simulink model "atrias_system_4khz"  (R2016b)
settings: Solver=FixedStepDiscrete  StartTime=0.0  StopTime=inf  FixedStep=elmo_sample_time  RelTol=1e-3
undefined symbols (not defined in the file or in its folder): gui_disable_cmd, gui_enable_cmd, gui_exit_cmd, gui_reset_cmd, HARD_MOTOR_POSITION_LIMITS_LOWER, HARD_MOTOR_POSITION_LIMITS_UPPER, HIP_ABS_MAX_ENCODER_TICKS, HIP_CURRENT_LIMIT, HIP_INC_MAX_ENCODER_TICKS, HIP_MOTOR_CONSTANT, HIP_MTR_GEAR_RATIO, HIP_MTR_MAX_TORQUE, LEFT_MOTOR_HIP_DIRECTION, LEG1_MOTOR_A_DIRECTION, LEG1_MOTOR_B_DIRECTION, LEG2_MOTOR_A_DIRECTION, LEG2_MOTOR_B_DIRECTION, LEG_CURRENT_LIMIT, LEG_INC_ENCODER_DIRECTION_LEFT_BACK, LEG_INC_ENCODER_DIRECTION_LEFT_FRONT, LEG_INC_ENCODER_DIRECTION_RIGHT_BACK, LEG_INC_ENCODER_DIRECTION_RIGHT_FRONT, LEG_INC_ENCODER_RAD_PER_TICK, LEG_MOTOR_CONSTANT, LEG_MTR_GEAR_RATIO, LEG_MTR_MAX_TORQUE, max_hip_velocity, max_motor_velocity, MEDULLA_ADC_MAX_VOLTS, MEDULLA_ADC_OFFSET_COUNTS, MEDULLA_STATE_ERROR, MEDULLA_STATE_HALT, MEDULLA_STATE_IDLE, MEDULLA_STATE_RESET, MEDULLA_STATE_RUN, MOTOR_POSITION_LIMITS_LOWER, MOTOR_POSITION_LIMITS_UPPER, MTR_HIP_MAX_CURRENT, MTR_MAX_CONT_CURRENT, MTR_MAX_COUNT, MTR_MAX_CURRENT, MTR_MAX_TEMP, RIGHT_MOTOR_HIP_DIRECTION
libraries: xpcethercatlib x190, simulink x37
(part 1 of 4)
settings Model: xpc_rtwmakecfg_data=_xpcethercatlib_  SimulationMode=external  ParamWorkspaceSource=ReferencedWorkspace  Creator=wmartin  LastModifiedBy=Will
settings SolverCC: EnableConcurrentExecution=on
settings DataIOCC: LimitDataPoints=on  MaxDataPoints=1000000000  SaveFormat=StructureWithTime  SaveOutput=off  SaveTime=off
settings OptimizationCC: BlockReduction=off  DefaultParameterBehavior=Inlined  OptimizeBlockIOStorage=off  BufferReuse=off  GlobalBufferReuse=off  ExpressionFolding=off  ExpressionDepthLimit=2147483647  LocalBlockOutputs=off  LifeSpan=inf  SimCompilerOptimization=on
settings DebuggingCC: UnderspecifiedInitializationDetection=Classic  MergeDetectMultiDrivingBlocksExec=none  SolverPrmCheckMsg=warning  StateNameClashWarn=warning  SFUnexpectedBacktrackingDiag=warning  SFNoUnconditionalDefaultTransitionDiag=warning  SFExecutionAtInitializationDiag=none
settings HardwareCC: ProdBitPerPointer=32  ProdBitPerSizeT=32  ProdBitPerPtrDiffT=32  ProdLargestAtomicFloat=None  ProdWordSize=32  ProdLongLongMode=on  ProdHWDeviceType=Generic->32-bit x86 compatible
settings ModelReferenceCC: EnableParallelModelReferenceBuilds=on  ModelReferenceNumInstancesAllowed=Single  ModelReferenceMinAlgLoopOccurrences=on  PropagateSignalLabelsOutOfModel=off
settings RTWCC: SystemTargetFile=slrt.tlc  TemplateMakefile=slrt_default_tmf  Description=Simulink Real-Time  RTWVerbose=off  RTWCompilerOptimization=on
settings CodeAppCC: MaxIdLength=256
settings SimulinkRealTimeCC: GeneratePreprocessorConditionals=Disable all  RL32LogBufSizeModifier=100000000
settings ConfigComp: CovMetricSettings=dw  CovHtmlReporting=on  CovSaveCumulativeToWorkspaceVar=on  CovSaveSingleToWorkspaceVar=on  CovExternalEMLEnable=off  CovSFcnEnable=off

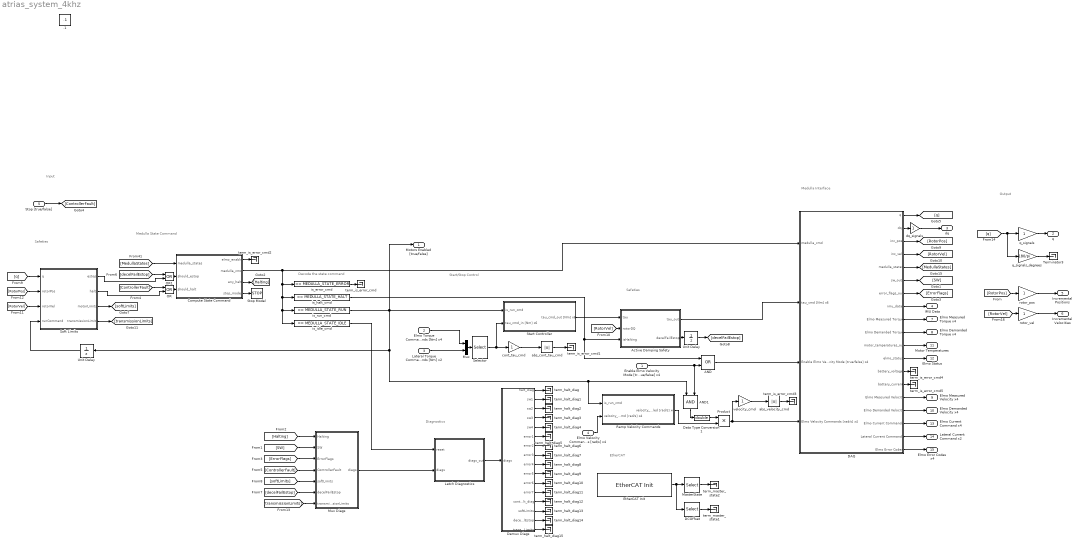
== system atrias_system_4khz ==
  note: Decode the state command
  note: Medulla Interface
  note: Medulla State Command
  note: Diagnostics
  note: EtherCAT
  note: Start/Stop Control
  note: Input
  note: Safeties
  note: Safeties
  note: Output
  Enable Elmo Velocity Mode [true/false] x4 : Inport  OutDataTypeStr=boolean  PortDimensions=4
  Elmo Torque Commands [Nm] x4 : Inport  Port=2  PortDimensions=4
  Lateral Torque Commands [Nm] x2 : Inport  Port=3  PortDimensions=2
  Elmo Velocity Commands [rad/s] x4 : Inport  Port=4  OutDataTypeStr=double  PortDimensions=4
  Stop [true/false] : Inport  Port=5  OutDataTypeStr=boolean
  AND : Logic  Operator=OR  AllPortsSameDT=off  OutDataTypeStr=boolean
  AND1 : Logic  AllPortsSameDT=off  OutDataTypeStr=boolean
  Active Damping Safety : MATLAB Function  TreatAsAtomicUnit=on
  Compute State Command : MATLAB Function  TreatAsAtomicUnit=on
  DAQ : Subsystem
  DCOffset : Selector  InputPortWidth=6  IndexOptions=Index vector (dialog)  Indices=[4]  OutputSizes=1
  Data Type Conversion1 : DataTypeConversion  OutDataTypeStr=double
  Demux Diags : MATLAB Function  TreatAsAtomicUnit=on
  EtherCAT Init : xpcethercatlib/EtherCAT Init   Priority=0  config_file=7medullas4emlos_09_19_2016_4khz.xml  device_id=0  pci_bus=2  pci_slot=0  dctuning=0  enaDebug=off  enaDC=on  errLink=off  masterDbg=off  stateChgDbg=off  baseClock=off  masterCfg=off  logFile='E:\dbglog.txt'  sample_time=0.000250  DCMode=2
  Latch Diagnostics : MATLAB Function  TreatAsAtomicUnit=on
  MasterState : Selector  InputPortWidth=6  IndexOptions=Index vector (dialog)  Indices=[2]  OutputSizes=1
  Mux : Mux  Inputs=2
  Mux Diags : MATLAB Function  TreatAsAtomicUnit=on
  OR : Logic  Operator=OR  AllPortsSameDT=off  OutDataTypeStr=boolean
  OR1 : Logic  Operator=OR  AllPortsSameDT=off  OutDataTypeStr=boolean
  Product : Product
  Ramp Velocity Commands : Subsystem
  Selector : Selector  InputPortWidth=6  IndexOptions=Index vector (dialog)  Indices=[1 2 5 3 4 6]  OutputSizes=1
  Soft Limits : MATLAB Function  TreatAsAtomicUnit=on
  Start Controller : Subsystem
  Stop Model : Stop
  Terminator3 : Terminator
  Unit Delay : UnitDelay  SampleTime=-1
  "Unit Delay " : UnitDelay  SampleTime=-1
  abs_cont_tau_cmd : Abs
  abs_velocity_cmd : Abs
  cont_tau_cmd : Gain
  dq_signals : Gain
  is_error_cmd : simulink/Logic and Bit Operations/Compare To Constant  relop===  const=MEDULLA_STATE_ERROR  OutDataTypeStr=boolean
  is_halt_cmd : simulink/Logic and Bit Operations/Compare To Constant  relop===  const=MEDULLA_STATE_HALT  OutDataTypeStr=boolean
  is_idle_cmd : simulink/Logic and Bit Operations/Compare To Constant  relop===  const=MEDULLA_STATE_IDLE  OutDataTypeStr=boolean
  is_run_cmd : simulink/Logic and Bit Operations/Compare To Constant  relop===  const=MEDULLA_STATE_RUN  OutDataTypeStr=boolean
  q_signals : Gain
  q_signals_degrees : Gain  Gain=180/pi
  rotor_pos : Gain
  rotor_vel : Gain
  term_halt_diag{,1..15} (16 alike) : Terminator
  term_is_error_cmd{,1..5} (6 alike) : Terminator
  term_master_state1 : Terminator
  term_master_state2 : Terminator
  velocity_cmd : Gain
  Motors Enabled [true/false] : Outport
  q : Outport  Port=2
  dq : Outport  Port=3
  IMU Data : Outport  Port=4
  Incremental Positions : Outport  Port=5
  Incremental Velocities : Outport  Port=6
  Elmo Measured Torque x4 : Outport  Port=7
  Elmo Demanded Torque x4 : Outport  Port=8
  Elmo Measured Velocity x4 : Outport  Port=9
  Elmo Demanded Velocity x4 : Outport  Port=10
  Motor Temperatures : Outport  Port=11
  Elmo Status : Outport  Port=12
  Elmo Current Command x4 : Outport  Port=13
  Lateral Current Command x2 : Outport  Port=14
  Elmo Error Codes x4 : Outport  Port=15
  .1 : Constant  IOType=siggen  Value=.1
  wires:
  [MedullaStates] -> Compute State Command/1(medulla_states)
  Compute State Command/3(any_halt) -> [Halting]
  Latch Diagnostics/1(diags_out) -> Demux Diags/1(diags)
  is_error_cmd/1 -> term_is_error_cmd/1
  Selector/1 -> Start Controller/2(tau_cmd_in [Nm] x6), cont_tau_cmd/1
  Start Controller/1(tau_cmd_out [Nm] x6) -> Active Damping Safety/1(tau)
  is_idle_cmd/1 -> Latch Diagnostics/1(reset)
  DAQ/6(sw_out) -> [SW]
  Mux Diags/1(diags) -> Latch Diagnostics/2(diags)
  [Halting] -> Mux Diags/1(Halting)
  [SW] -> Mux Diags/2(SW)
  Demux Diags/2(sw1) -> term_halt_diag1/1
  Demux Diags/5(sw4) -> term_halt_diag4/1
  Demux Diags/4(sw3) -> term_halt_diag3/1
  Demux Diags/3(sw2) -> term_halt_diag2/1
  DAQ/7(error_flags_out) -> [ErrorFlags]
  [ErrorFlags] -> Mux Diags/3(ErrorFlags)
  Demux Diags/1(halt_diag) -> term_halt_diag/1
  Demux Diags/12(error7) -> term_halt_diag11/1
  Demux Diags/11(error6) -> term_halt_diag10/1
  Demux Diags/10(error5) -> term_halt_diag9/1
  Demux Diags/9(error4) -> term_halt_diag8/1
  Demux Diags/8(error3) -> term_halt_diag7/1
  Demux Diags/7(error2) -> term_halt_diag6/1
  Demux Diags/6(error1) -> term_halt_diag5/1
  abs_cont_tau_cmd/1 -> term_is_error_cmd1/1
  DAQ/8(imu_data) -> IMU Data/1
  [ControllerFault] -> Mux Diags/4(ControllerFault)
  Demux Diags/13(contrlr_fault_diag) -> term_halt_diag12/1
  [RotorPos] -> Soft Limits/2(rotorPos)
  [RotorVel] -> Soft Limits/3(rotorVel)
  EtherCAT Init/1 -> DCOffset/1, MasterState/1
  cont_tau_cmd/1 -> abs_cont_tau_cmd/1
  Stop [true/false]/1 -> [ControllerFault]
  [softLimits] -> Mux Diags/5(softLimits)
  Demux Diags/14(softLimits) -> term_halt_diag13/1
  Soft Limits/3(motorLimits) -> [softLimits]
  is_run_cmd/1 -> Start Controller/1(is_run_cmd), Motors Enabled [true/false]/1, Ramp Velocity Commands/1(is_run_cmd), AND1/1, Unit Delay/1
  Active Damping Safety/1(tau_out) -> DAQ/2(tau_cmd [Nm] x6)
  [RotorVel] -> Active Damping Safety/2(rotorDQ)
  DCOffset/1 -> term_master_state1/1
  [q] -> Soft Limits/1(q)
  [decelFailEstop] -> Mux Diags/6(decelFailEstop)
  Demux Diags/15(decelFailEstop) -> term_halt_diag14/1
  DAQ/5(medulla_states) -> [MedullaStates]
  Active Damping Safety/2(decelFailEstop) -> "Unit Delay "/1
  "Unit Delay "/1 -> [decelFailEstop]
  DAQ/9(Elmo Measured Torque) -> Elmo Measured Torque x4/1
  [ControllerFault] -> OR/1
  Soft Limits/2(halt) -> OR/2
  OR/1 -> Compute State Command/3(should_halt)
  Unit Delay/1 -> Soft Limits/4(runCommand)
  [decelFailEstop] -> OR1/1
  OR1/1 -> Compute State Command/2(should_estop)
  Soft Limits/1(estop) -> OR1/2
  Soft Limits/4(transmissionLimits) -> [transmissionLimits]
  [transmissionLimits] -> Mux Diags/7(transmissionLimits)
  Demux Diags/16(transmissionLimits) -> term_halt_diag15/1
  DAQ/11(motor_temperatures_out) -> Motor Temperatures/1
  q_signals_degrees/1 -> Terminator3/1
  rotor_pos/1 -> Incremental Positions/1
  Compute State Command/2(medulla_cmd) -> is_idle_cmd/1, is_run_cmd/1, is_halt_cmd/1, is_error_cmd/1, DAQ/1(medulla_cmd)
  Compute State Command/1(elmo_enable) -> term_is_error_cmd2/1
  DAQ/12(elmo_status) -> Elmo Status/1
  MasterState/1 -> term_master_state2/1
  DAQ/4(inc_vel) -> [RotorVel]
  [RotorVel] -> rotor_vel/1
  rotor_vel/1 -> Incremental Velocities/1
  DAQ/3(inc_pos) -> [RotorPos]
  [RotorPos] -> rotor_pos/1
  dq_signals/1 -> dq/1
  DAQ/2(dq) -> dq_signals/1
  DAQ/1(q) -> [q]
  [q] -> q_signals/1, q_signals_degrees/1
  q_signals/1 -> q/1
  Compute State Command/4(stop_model) -> Stop Model/1
  Enable Elmo Velocity Mode [true/false] x4/1 -> AND1/2, AND/2
  is_halt_cmd/1 -> AND/1, Active Damping Safety/3(isHalting)
  Ramp Velocity Commands/1(velocity_cmd_scaled [rad/s] x4) -> Product/2
  Data Type Conversion1/1 -> Product/1
  AND1/1 -> Data Type Conversion1/1
  DAQ/15(Elmo Measured Velocity) -> Elmo Measured Velocity x4/1
  DAQ/17(Elmo Current Commands) -> Elmo Current Command x4/1
  DAQ/18(Lateral Current Commands) -> Lateral Current Command x2/1
  DAQ/10(Elmo Demanded Torque) -> Elmo Demanded Torque x4/1
  Elmo Velocity Commands [rad/s] x4/1 -> Ramp Velocity Commands/2(velocity_cmd [rad/s] x4)
  Product/1 -> velocity_cmd/1, DAQ/4(Elmo Velocity Commands [rad/s] x4)
  abs_velocity_cmd/1 -> term_is_error_cmd3/1
  AND/1 -> DAQ/3(Enable Elmo Velocity Mode [true/false] x4)
  velocity_cmd/1 -> abs_velocity_cmd/1
  DAQ/19(Elmo Error Codes) -> Elmo Error Codes x4/1
  DAQ/16(Elmo Demanded Velocity) -> Elmo Demanded Velocity x4/1
  DAQ/13(battery_voltage) -> term_is_error_cmd4/1
  DAQ/14(battery_current) -> term_is_error_cmd5/1
  Lateral Torque Commands [Nm] x2/1 -> Mux/2
  Elmo Torque Commands [Nm] x4/1 -> Mux/1
  Mux/1 -> Selector/1

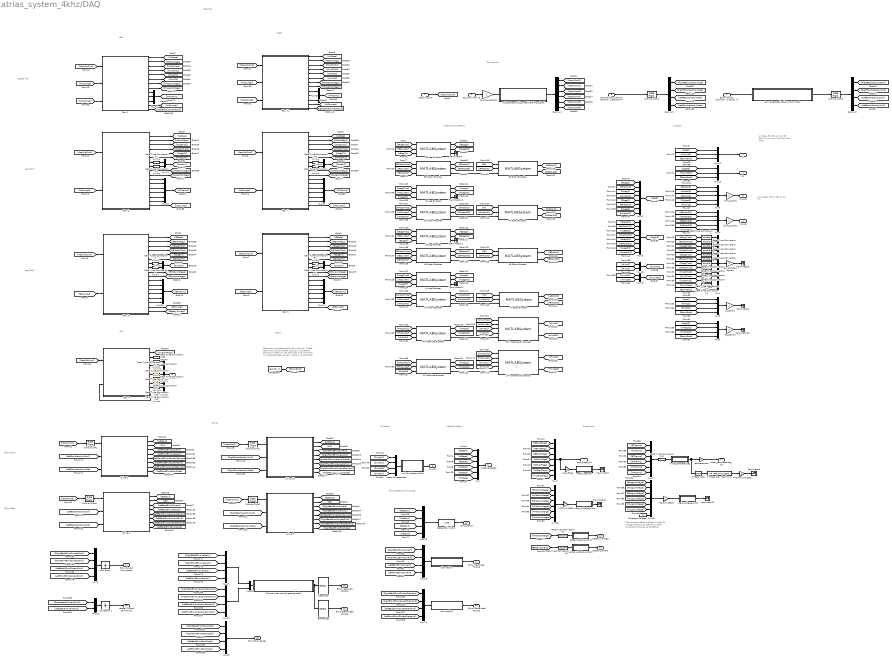
== system atrias_system_4khz/DAQ ==
  note: Fake boom encoder signals for q and dq.
      | These keep q and dq the same size as it was
      | before the boom medulla was removed.
      | The IMU block will replace these values if
      | used by a controller
  note: The constant fakes the boom medulla
      | voltage reading to keep the vector
      | dimensions the same as before.
  note: Left
  note: Right
  note: Lateral Hip
  note: Leg Back
  note: Leg Front
  note: Medullas
  note: Angle Computations
  note: Commands
  note: Switches
  note: Supervisory
  note: q Order:
      |
      | rBl
      | rBm
      | rAl
      | rAm
      |
      | lBl
      | lBm
      | lAl
      | lAm
      |
      | rHm
      | lHm
      |
      | Roll
      | Yaw
      | Pitch
  note: Medulla States
  note: IMU
  note: Elmos
  note: Elmo Front
  note: Elmo Back
  note: Elmo States and Torques
  note: qinc Order:
      |
      | rBr
      | rAr
      | lBr
      | lAr
      |
      | rHr
      | lHr
  note: Boom
  note: Outputs
  medulla_cmd : Inport
  tau_cmd [Nm] x6 : Inport  Port=2  OutDataTypeStr=double  PortDimensions=6
  Enable Elmo Velocity Mode [true/false] x4 : Inport  Port=3
  Elmo Velocity Commands [rad/s] x4 : Inport  Port=4
  1kHz to 2kHz{,1..5} (6 alike) : RateTransition  OutPortSampleTime=elmo_sample_time
  Box 1 : Subsystem
  Box 11 : Subsystem
  Box 4 : Subsystem
  Box 5 : Subsystem
  Box 6 : Subsystem
  Box 7 : Subsystem
  Box 8 : Subsystem
  Conversion : Subsystem
  Conversion1 : Subsystem
  Convert geared rad/s to rotor cnts/s : Subsystem
  Convert rotor cnt/s to geared rad/s : Subsystem
  Data Type Conversion{1..16,27..28,51..52,75..76,112..121} (32 alike) : DataTypeConversion  OutDataTypeStr=double
  Demanded : Selector  InputPortWidth=8  IndexOptions=Index vector (dialog)  Indices=[5 6 7 8]  OutputSizes=1
  Demux1 : Demux  Outputs=6
  Demux2 : Demux
  Demux3 : Demux
  Drive 10 : Subsystem
  Drive 2 : Subsystem
  Drive 3 : Subsystem
  Drive 9 : Subsystem
  FakeBoom : Constant  Value=zeros(3, 1)
  FakeLogicVoltage : Constant  Value=0  OutDataTypeStr=uint16
  Hottest Motor : MinMax  Function=max
  If Hotter than Maximum : simulink/Logic and Bit Operations/Compare To Constant  relop=>=  const=MTR_MAX_TEMP  OutDataTypeStr=boolean
  LA Leg Encoder : MATLABSystem  System=AbsEncoder  unitsPerTick=LEG2_LEG_B_RAD_PER_CNT  calibTicks=LEG2_LEG_B_CALIB_VAL  calibVal=LEG_B_CALIB_LOC  unwrapMod=0  dropRepeatVals=true  minPos=HARD_MOTOR_POSITION_LIMITS_LOWER(1) - .5  maxPos=HARD_MOTOR_POSITION_LIMITS_UPPER(1) + .5  maxSpd=2 * max_motor_velocity  sample_time=sample_time  counterMod=256  medullaFreq=MEDULLA_TIMER_FREQ  initPosOut=0  initVelOut=0  checkInf=true  calibOnce=true  SimulateUsing=Code generation
      mask Type: AbsEncoder
      mask Display:
      | disp('AbsEncoder');
      | port_label('input',1,'ticks');
      | port_label('input',2,'counter');
      | port_label('input',3,'timestamp');
      | port_label('output',1,'pos');
      | port_label('output',2,'vel');
      | port_label('output',3,'isValid');
  LA Motor Encoder : MATLABSystem  System=AbsEncoder  unitsPerTick=LEG2_TRAN_B_RAD_PER_CNT  calibTicks=LEG2_TRAN_B_CALIB_VAL  calibVal=LEG_B_CALIB_LOC  unwrapMod=0  dropRepeatVals=true  minPos=HARD_MOTOR_POSITION_LIMITS_LOWER(1) - .5  maxPos=HARD_MOTOR_POSITION_LIMITS_UPPER(1) + .5  maxSpd=2 * max_motor_velocity  sample_time=sample_time  counterMod=256  medullaFreq=MEDULLA_TIMER_FREQ  initPosOut=0  initVelOut=0  checkInf=true  calibOnce=true  SimulateUsing=Code generation
      mask Type: AbsEncoder
      mask Display:
      | disp('AbsEncoder');
      | port_label('input',1,'ticks');
      | port_label('input',2,'counter');
      | port_label('input',3,'timestamp');
      | port_label('output',1,'pos');
      | port_label('output',2,'vel');
      | port_label('output',3,'isValid');
  LA Rotor Encoder : MATLABSystem  System=ElmoIncremental  unitsPerTick=LEG_INC_ENCODER_DIRECTION_LEFT_FRONT*LEG_INC_ENCODER_RAD_PER_TICK  sample_time=elmo_sample_time  initPosOut=0  initVelOut=0  checkInf=false  calibOnce=true  SimulateUsing=Code generation
      mask Type: ElmoIncremental
      mask Display:
      | disp('ElmoIncremental');
      | port_label('input',1,'incTicks');
      | port_label('input',2,'calibVal');
      | port_label('input',3,'calibTrig');
      | port_label('output',1,'pos');
      | port_label('output',2,'vel');
  LB Leg Encoder : MATLABSystem  System=AbsEncoder  unitsPerTick=LEG2_LEG_A_RAD_PER_CNT  calibTicks=LEG2_LEG_A_CALIB_VAL  calibVal=LEG_A_CALIB_LOC  unwrapMod=0  dropRepeatVals=true  minPos=HARD_MOTOR_POSITION_LIMITS_LOWER(2) - .5  maxPos=HARD_MOTOR_POSITION_LIMITS_UPPER(2) + .5  maxSpd=2 * max_motor_velocity  sample_time=sample_time  counterMod=256  medullaFreq=MEDULLA_TIMER_FREQ  initPosOut=0  initVelOut=0  checkInf=true  calibOnce=true  SimulateUsing=Code generation
      mask Type: AbsEncoder
      mask Display:
      | disp('AbsEncoder');
      | port_label('input',1,'ticks');
      | port_label('input',2,'counter');
      | port_label('input',3,'timestamp');
      | port_label('output',1,'pos');
      | port_label('output',2,'vel');
      | port_label('output',3,'isValid');
  LB Motor Encoder : MATLABSystem  System=AbsEncoder  unitsPerTick=LEG2_TRAN_A_RAD_PER_CNT  calibTicks=LEG2_TRAN_A_CALIB_VAL  calibVal=LEG_A_CALIB_LOC  unwrapMod=0  dropRepeatVals=true  minPos=HARD_MOTOR_POSITION_LIMITS_LOWER(2) - .5  maxPos=HARD_MOTOR_POSITION_LIMITS_UPPER(2) + .5  maxSpd=2 * max_motor_velocity  sample_time=sample_time  counterMod=256  medullaFreq=MEDULLA_TIMER_FREQ  initPosOut=0  initVelOut=0  checkInf=true  calibOnce=true  SimulateUsing=Code generation
      mask Type: AbsEncoder
      mask Display:
      | disp('AbsEncoder');
      | port_label('input',1,'ticks');
      | port_label('input',2,'counter');
      | port_label('input',3,'timestamp');
      | port_label('output',1,'pos');
      | port_label('output',2,'vel');
      | port_label('output',3,'isValid');
  LB Rotor Encoder : MATLABSystem  System=ElmoIncremental  unitsPerTick=LEG_INC_ENCODER_DIRECTION_LEFT_BACK*LEG_INC_ENCODER_RAD_PER_TICK  sample_time=elmo_sample_time  initPosOut=0  initVelOut=0  checkInf=false  calibOnce=true  SimulateUsing=Code generation
      mask Type: ElmoIncremental
      mask Display:
      | disp('ElmoIncremental');
      | port_label('input',1,'incTicks');
      | port_label('input',2,'calibVal');
      | port_label('input',3,'calibTrig');
      | port_label('output',1,'pos');
      | port_label('output',2,'vel');
  LH Absolute Encoder : MATLABSystem  System=AbsEncoder  unitsPerTick=LEFT_HIP_ABS_ENCODER_RAD_PER_TICK  calibTicks=LEFT_HIP_CALIB_VAL  calibVal=LEFT_HIP_CALIB_POS  unwrapMod=HIP_ABS_MAX_ENCODER_TICKS+1  dropRepeatVals=false  minPos=-.5  maxPos=.3  maxSpd=2 * max_hip_velocity  sample_time=sample_time  counterMod=256  medullaFreq=MEDULLA_TIMER_FREQ  initPosOut=0  initVelOut=0  checkInf=true  calibOnce=true  SimulateUsing=Code generation
      mask Type: AbsEncoder
      mask Display:
      | disp('AbsEncoder');
      | port_label('input',1,'ticks');
      | port_label('input',2,'counter');
      | port_label('input',3,'timestamp');
      | port_label('output',1,'pos');
      | port_label('output',2,'vel');
      | port_label('output',3,'isValid');
  LH Incremental Encoder : MATLABSystem  System=IncEncoder  unitsPerTick=LEFT_HIP_INC_ENCODER_RAD_PER_TICK  unwrapMod=HIP_INC_MAX_ENCODER_TICKS+1  sample_time=sample_time  counterMod=256  medullaFreq=MEDULLA_TIMER_FREQ  initPosOut=0  initVelOut=0  checkInf=true  calibOnce=true  SimulateUsing=Code generation
      mask Type: IncEncoder
      mask Display:
      | disp('IncEncoder');
      | port_label('input',1,'ticks');
      | port_label('input',2,'counter');
      | port_label('input',3,'timestamp');
      | port_label('input',4,'absPos');
      | port_label('input',5,'absIsValid');
      | port_label('output',1,'pos');
      | port_label('output',2,'vel');
  Limit Switches to Bool : MATLAB Function  TreatAsAtomicUnit=on
  Measured : Selector  InputPortWidth=8  IndexOptions=Index vector (dialog)  Indices=[1 2 3 4]  OutputSizes=1
  Mux{,17,21,27,32..33,36} (7 alike) : Mux  Inputs=6
  Mux1 : Mux  Inputs=13
  Mux{10,15,31,34} (4 alike) : Mux  Inputs=3
  Mux{11..14,16,18,20,29} (8 alike) : Mux  Inputs=2
  Mux{2,8..9,19,22..25,28} (9 alike) : Mux
  Mux26 : Mux  Inputs=9
  Mux3 : Mux  Inputs=5
  Mux35 : Mux  Inputs=7
  Mux4 : Mux  Inputs=5
  Mux5 : Mux  Inputs=8
  Mux6 : Mux  Inputs=8
  Mux7 : Mux  Inputs=7
  RA Leg Encoder : MATLABSystem  System=AbsEncoder  unitsPerTick=LEG1_LEG_B_RAD_PER_CNT  calibTicks=LEG1_LEG_B_CALIB_VAL  calibVal=LEG_B_CALIB_LOC  unwrapMod=0  dropRepeatVals=true  minPos=HARD_MOTOR_POSITION_LIMITS_LOWER(1) - .5  maxPos=HARD_MOTOR_POSITION_LIMITS_UPPER(1) + .5  maxSpd=2 * max_motor_velocity  sample_time=sample_time  counterMod=256  medullaFreq=MEDULLA_TIMER_FREQ  initPosOut=0  initVelOut=0  checkInf=true  calibOnce=true  SimulateUsing=Code generation
      mask Type: AbsEncoder
      mask Display:
      | disp('AbsEncoder');
      | port_label('input',1,'ticks');
      | port_label('input',2,'counter');
      | port_label('input',3,'timestamp');
      | port_label('output',1,'pos');
      | port_label('output',2,'vel');
      | port_label('output',3,'isValid');
  RA Motor Encoder : MATLABSystem  System=AbsEncoder  unitsPerTick=LEG1_TRAN_B_RAD_PER_CNT  calibTicks=LEG1_TRAN_B_CALIB_VAL  calibVal=LEG_B_CALIB_LOC  unwrapMod=0  dropRepeatVals=true  minPos=HARD_MOTOR_POSITION_LIMITS_LOWER(1) - .5  maxPos=HARD_MOTOR_POSITION_LIMITS_UPPER(1) + .5  maxSpd=2 * max_motor_velocity  sample_time=sample_time  counterMod=256  medullaFreq=MEDULLA_TIMER_FREQ  initPosOut=0  initVelOut=0  checkInf=true  calibOnce=true  SimulateUsing=Code generation
      mask Type: AbsEncoder
      mask Display:
      | disp('AbsEncoder');
      | port_label('input',1,'ticks');
      | port_label('input',2,'counter');
      | port_label('input',3,'timestamp');
      | port_label('output',1,'pos');
      | port_label('output',2,'vel');
      | port_label('output',3,'isValid');
  RA Rotor Encoder : MATLABSystem  System=ElmoIncremental  unitsPerTick=LEG_INC_ENCODER_DIRECTION_RIGHT_FRONT*LEG_INC_ENCODER_RAD_PER_TICK  sample_time=elmo_sample_time  initPosOut=0  initVelOut=0  checkInf=false  calibOnce=true  SimulateUsing=Code generation
      mask Type: ElmoIncremental
      mask Display:
      | disp('ElmoIncremental');
      | port_label('input',1,'incTicks');
      | port_label('input',2,'calibVal');
      | port_label('input',3,'calibTrig');
      | port_label('output',1,'pos');
      | port_label('output',2,'vel');
  RB Leg Encoder : MATLABSystem  System=AbsEncoder  unitsPerTick=LEG1_LEG_A_RAD_PER_CNT  calibTicks=LEG1_LEG_A_CALIB_VAL  calibVal=LEG_A_CALIB_LOC  unwrapMod=0  dropRepeatVals=true  minPos=HARD_MOTOR_POSITION_LIMITS_LOWER(2) - .5  maxPos=HARD_MOTOR_POSITION_LIMITS_UPPER(2) + .5  maxSpd=2 * max_motor_velocity  sample_time=sample_time  counterMod=256  medullaFreq=MEDULLA_TIMER_FREQ  initPosOut=0  initVelOut=0  checkInf=true  calibOnce=true  SimulateUsing=Code generation
      mask Type: AbsEncoder
      mask Display:
      | disp('AbsEncoder');
      | port_label('input',1,'ticks');
      | port_label('input',2,'counter');
      | port_label('input',3,'timestamp');
      | port_label('output',1,'pos');
      | port_label('output',2,'vel');
      | port_label('output',3,'isValid');
  RB Motor Encoder : MATLABSystem  System=AbsEncoder  unitsPerTick=LEG1_TRAN_A_RAD_PER_CNT  calibTicks=LEG1_TRAN_A_CALIB_VAL  calibVal=LEG_A_CALIB_LOC  unwrapMod=0  dropRepeatVals=true  minPos=HARD_MOTOR_POSITION_LIMITS_LOWER(2) - .5  maxPos=HARD_MOTOR_POSITION_LIMITS_UPPER(2) + .5  maxSpd=2 * max_motor_velocity  sample_time=sample_time  counterMod=256  medullaFreq=MEDULLA_TIMER_FREQ  initPosOut=0  initVelOut=0  checkInf=true  calibOnce=true  SimulateUsing=Code generation
      mask Type: AbsEncoder
      mask Display:
      | disp('AbsEncoder');
      | port_label('input',1,'ticks');
      | port_label('input',2,'counter');
      | port_label('input',3,'timestamp');
      | port_label('output',1,'pos');
      | port_label('output',2,'vel');
      | port_label('output',3,'isValid');
  RB Rotor Encoder : MATLABSystem  System=ElmoIncremental  unitsPerTick=LEG_INC_ENCODER_DIRECTION_RIGHT_BACK*LEG_INC_ENCODER_RAD_PER_TICK  sample_time=elmo_sample_time  initPosOut=0  initVelOut=0  checkInf=false  calibOnce=true  SimulateUsing=Code generation
      mask Type: ElmoIncremental
      mask Display:
      | disp('ElmoIncremental');
      | port_label('input',1,'incTicks');
      | port_label('input',2,'calibVal');
      | port_label('input',3,'calibTrig');
      | port_label('output',1,'pos');
      | port_label('output',2,'vel');
  RH Absolute Encoder : MATLABSystem  System=AbsEncoder  unitsPerTick=RIGHT_HIP_ABS_ENCODER_RAD_PER_TICK  calibTicks=RIGHT_HIP_CALIB_VAL  calibVal=RIGHT_HIP_CALIB_POS  unwrapMod=HIP_ABS_MAX_ENCODER_TICKS+1  dropRepeatVals=false  minPos=-.5  maxPos=.3  maxSpd=2 * max_hip_velocity  sample_time=sample_time  counterMod=256  medullaFreq=MEDULLA_TIMER_FREQ  initPosOut=0  initVelOut=0  checkInf=true  calibOnce=true  SimulateUsing=Code generation
      mask Type: AbsEncoder
      mask Display:
      | disp('AbsEncoder');
      | port_label('input',1,'ticks');
      | port_label('input',2,'counter');
      | port_label('input',3,'timestamp');
      | port_label('output',1,'pos');
      | port_label('output',2,'vel');
      | port_label('output',3,'isValid');
  RH Incremental Encoder : MATLABSystem  System=IncEncoder  unitsPerTick=RIGHT_HIP_INC_ENCODER_RAD_PER_TICK  unwrapMod=HIP_INC_MAX_ENCODER_TICKS+1  sample_time=sample_time  counterMod=256  medullaFreq=MEDULLA_TIMER_FREQ  initPosOut=0  initVelOut=0  checkInf=true  calibOnce=true  SimulateUsing=Code generation
      mask Type: IncEncoder
      mask Display:
      | disp('IncEncoder');
      | port_label('input',1,'ticks');
      | port_label('input',2,'counter');
      | port_label('input',3,'timestamp');
      | port_label('input',4,'absPos');
      | port_label('input',5,'absIsValid');
      | port_label('output',1,'pos');
      | port_label('output',2,'vel');
  States Dbl->Uint1 : DataTypeConversion  OutDataTypeStr=uint8
  Terminator{1,4..8,10..14} (11 alike) : Terminator
  Thermal_Indicator : Gain
  "Unit Delay " : UnitDelay  SampleTime=-1
  Unit Delay 1 : UnitDelay  SampleTime=-1
  Vector Concatenate : Concatenate  NumInputs=4
  battery_ADC_to_current : MATLAB Function  TreatAsAtomicUnit=on
  battery_ADC_to_volts : MATLAB Function  TreatAsAtomicUnit=on
  dq_signals : Gain
  dqinc_signals : Gain
  error_flags : Gain  OutDataTypeStr=double
  logic_voltage_volts : MATLAB Function  TreatAsAtomicUnit=on
  logic_voltages : Gain  OutDataTypeStr=double
  medulla_errors : MATLAB Function  TreatAsAtomicUnit=on
  motor_temperatures : MATLAB Function  TreatAsAtomicUnit=on
  motor_voltage_volts : MATLAB Function  TreatAsAtomicUnit=on
  motor_voltages : Gain  OutDataTypeStr=double
  mtr_torque_cmd_to_medulla/elmo_signal : Subsystem
  q_signals : Gain
  qinc_signals : Gain
  raw_encoder_signals : Gain
  tau_cmd_signals : Gain
  temperatures : Gain
  q : Outport
  dq : Outport  Port=2
  inc_pos : Outport  Port=3
  inc_vel : Outport  Port=4
  medulla_states : Outport  Port=5  OutDataTypeStr=uint8
  sw_out : Outport  Port=6
  error_flags_out : Outport  Port=7  OutDataTypeStr=uint8
  imu_data : Outport  Port=8
  Elmo Measured Torque : Outport  Port=9
  Elmo Demanded Torque : Outport  Port=10
  motor_temperatures_out : Outport  Port=11
  elmo_status : Outport  Port=12
  battery_voltage : Outport  Port=13
  battery_current : Outport  Port=14
  Elmo Measured Velocity : Outport  Port=15
  Elmo Demanded Velocity : Outport  Port=16
  Elmo Current Commands : Outport  Port=17
  Lateral Current Commands : Outport  Port=18
  Elmo Error Codes : Outport  Port=19
  wires:
  mtr_torque_cmd_to_medulla/elmo_signal/1(current_cmd) -> Demux1/1
  Data Type Conversion27/1 -> Mux14/1
  Data Type Conversion2/1 -> Mux13/1
  tau_cmd [Nm] x6/1 -> tau_cmd_signals/1
  Data Type Conversion75/1 -> Mux11/1
  Data Type Conversion51/1 -> Mux12/1
  Demux1/1 -> [MotorCmd1]
  Demux1/2 -> [MotorCmd2]
  Demux1/3 -> [MotorCmd3]
  Demux1/4 -> [MotorCmd4]
  Demux1/5 -> [MotorCmd5]
  Demux1/6 -> [MotorCmd6]
  tau_cmd_signals/1 -> mtr_torque_cmd_to_medulla/elmo_signal/1(tau_cmd [Nm] x6)
  motor_voltage_volts/1(volt) -> Terminator6/1
  medulla_errors/1(errors) -> Terminator7/1
  logic_voltage_volts/1(volt) -> Terminator12/1
  medulla_cmd/1 -> [MedullaCmd]
  [Switch1] -> Vector Concatenate/1
  [Switch2] -> Vector Concatenate/2
  [Switch3] -> Vector Concatenate/3
  [Switch4] -> Vector Concatenate/4
  Vector Concatenate/1 -> Limit Switches to Bool/1(sw)
  Limit Switches to Bool/1(sw_out) -> sw_out/1
  Mux7/1 -> error_flags/1, error_flags_out/1
  Box 4/4(RotationZ) -> Data Type Conversion114/1
  Box 4/5(AccelerationX) -> Data Type Conversion115/1
  Box 4/6(AccelerationY) -> Data Type Conversion116/1
  Box 4/7(AccelerationZ) -> Data Type Conversion117/1
  Data Type Conversion112/1 -> Mux26/1
  Data Type Conversion113/1 -> Mux26/2
  Data Type Conversion114/1 -> Mux26/3
  Box 4/1(ErrorFlags) -> [imuErrorFlags]
  Data Type Conversion117/1 -> Mux26/6
  Data Type Conversion116/1 -> Mux26/5
  Data Type Conversion115/1 -> Mux26/4
  Mux26/1 -> imu_data/1
  [MedullaCmd] -> Box 4/1(MedullaCmd)
  [rBStatus] -> Mux28/1
  States Dbl->Uint1/1 -> elmo_status/1
  Mux28/1 -> States Dbl->Uint1/1
  [rAStatus] -> Mux28/2
  [lBStatus] -> Mux28/3
  [lAStatus] -> Mux28/4
  Box 1/1(State) -> [lHState]
  Box 1/2(ErrorFlags) -> [lHErrorFlags]
  Box 1/7(MotorVoltage) -> [lHMotorVoltage]
  Box 1/8(LogicVoltage) -> [lHLogicVoltage]
  Box 1/9(Thermistor0) -> Mux34/1
  Box 1/10(Thermistor1) -> Mux34/2
  Box 1/11(Thermistor2) -> Mux34/3
  [MedullaCmd] -> Box 1/1(MedullaCmd)
  [MotorCmd6] -> Box 1/3(MotorCmd)
  [MedullaCmd] -> Box 11/1(MedullaCmd)
  [MotorCmd5] -> Box 11/3(MotorCmd)
  Box 11/1(State) -> [rHState]
  Box 11/2(ErrorFlags) -> [rHErrorFlags]
  Box 11/7(MotorVoltage) -> [rHMotorVoltage]
  Box 11/8(LogicVoltage) -> [rHLogicVoltage]
  Box 11/9(Thermistor0) -> Mux31/1
  Box 11/10(Thermistor1) -> Mux31/2
  Box 11/11(Thermistor2) -> Mux31/3
  Box 5/7(ToeSensor) -> Data Type Conversion2/1
  Box 5/8(LimitSwitch) -> Data Type Conversion4/1
  Box 5/1(State) -> [lBState]
  Box 5/2(ErrorFlags) -> [lBErrorFlags]
  Box 5/9(MotorVoltage) -> [lBMotorVoltage]
  Box 5/10(LogicVoltage) -> [lBLogicVoltage]
  Box 5/11(Thermistor0) -> Mux32/1
  Box 5/12(Thermistor1) -> Mux32/2
  Box 5/13(Thermistor2) -> Mux32/3
  Box 5/14(Thermistor3) -> Mux32/4
  Box 5/15(Thermistor4) -> Mux32/5
  Box 5/16(Thermistor5) -> Mux32/6
  [MedullaCmd] -> Box 5/1(MedullaCmd)
  Box 5/17(Counter) -> [lBCounter]
  [MotorCmd3] -> 1kHz to 2kHz3/1
  Drive 3/1(status) -> [lBStatus]
  [MotorCmd1] -> 1kHz to 2kHz2/1
  Drive 9/1(status) -> [rBStatus]
  [MotorCmd4] -> 1kHz to 2kHz/1
  Drive 2/1(status) -> [lAStatus]
  Data Type Conversion76/1 -> Mux11/2
  Mux11/1 -> [Switch2]
  Data Type Conversion52/1 -> Mux12/2
  Mux12/1 -> [Switch1]
  Data Type Conversion4/1 -> Mux13/2
  Mux13/1 -> [Switch3]
  Data Type Conversion28/1 -> Mux14/2
  Mux14/1 -> [Switch4]
  error_flags/1 -> medulla_errors/1(u)
  logic_voltages/1 -> logic_voltage_volts/1(u)
  motor_voltages/1 -> motor_voltage_volts/1(u)
  Drive 3/2(rotor_tics) -> [lBr]
  Drive 9/2(rotor_tics) -> [rBr]
  Drive 9/3(ElmoCurrent) -> [RightBackElmoCurrent]
  Drive 2/3(ElmoCurrent) -> [LeftFrontElmoCurrent]
  Drive 3/3(ElmoCurrent) -> [LeftBackElmoCurrent]
  [RightBackElmoCurrent] -> Mux25/1
  [RightFrontElmoCurrent] -> Mux25/2
  [LeftBackElmoCurrent] -> Mux25/3
  [LeftFrontElmoCurrent] -> Mux25/4
  Mux25/1 -> Conversion/1(Elmo Current)
  Conversion/1(Torque) -> Elmo Measured Torque/1
  motor_temperatures/1(temp) -> Hottest Motor/1, temperatures/1
  temperatures/1 -> motor_temperatures_out/1
  [MedullaCmd] -> Box 6/1(MedullaCmd)
  Box 6/17(Counter) -> [lACounter]
  Box 6/7(ToeSensor) -> Data Type Conversion27/1
  Box 6/8(LimitSwitch) -> Data Type Conversion28/1
  Box 6/1(State) -> [lAState]
  Box 6/2(ErrorFlags) -> [lAErrorFlags]
  Box 6/9(MotorVoltage) -> [lAMotorVoltage]
  Box 6/10(LogicVoltage) -> [lALogicVoltage]
  Box 6/11(Thermistor0) -> Mux33/1
  Box 6/12(Thermistor1) -> Mux33/2
  Box 6/13(Thermistor2) -> Mux33/3
  Box 6/14(Thermistor3) -> Mux33/4
  Box 6/15(Thermistor4) -> Mux33/5
  Box 6/16(Thermistor5) -> Mux33/6
  [MedullaCmd] -> Box 7/1(MedullaCmd)
  Box 7/17(Counter) -> [rACounter]
  Box 7/7(ToeSensor) -> Data Type Conversion75/1
  Box 7/8(LimitSwitch) -> Data Type Conversion76/1
  Box 7/1(State) -> [rAState]
  Box 7/9(MotorVoltage) -> [rAMotorVoltage]
  Box 7/10(LogicVoltage) -> [rALogicVoltage]
  Box 7/11(Thermistor0) -> Mux27/1
  Box 7/12(Thermistor1) -> Mux27/2
  Box 7/13(Thermistor2) -> Mux27/3
  Box 7/14(Thermistor3) -> Mux27/4
  Box 7/15(Thermistor4) -> Mux27/5
  Box 7/16(Thermistor5) -> Mux27/6
  [MedullaCmd] -> Box 8/1(MedullaCmd)
  Box 8/17(Counter) -> [rBCounter]
  Box 8/7(ToeSensor) -> Data Type Conversion51/1
  Box 8/8(LimitSwitch) -> Data Type Conversion52/1
  Box 8/1(State) -> [rBState]
  Box 8/2(ErrorFlags) -> [rBErrorFlags]
  Box 8/9(MotorVoltage) -> [rBMotorVoltage]
  Box 8/10(LogicVoltage) -> [rBLogicVoltage]
  Box 8/11(Thermistor0) -> Mux21/1
  Box 8/12(Thermistor1) -> Mux21/2
  Box 8/13(Thermistor2) -> Mux21/3
  Box 8/14(Thermistor3) -> Mux21/4
  Box 8/15(Thermistor4) -> Mux21/5
  Box 8/16(Thermistor5) -> Mux21/6
  [MotorCmd2] -> 1kHz to 2kHz1/1
  Drive 10/1(status) -> [rAStatus]
  Drive 10/3(ElmoCurrent) -> [RightFrontElmoCurrent]
  Box 4/8(Sequence) -> Data Type Conversion118/1
  Data Type Conversion118/1 -> Mux26/7
  Box 4/9(Status) -> Data Type Conversion120/1
  Box 4/2(RotationX) -> Data Type Conversion112/1
  Box 4/3(RotationY) -> Data Type Conversion113/1
  Data Type Conversion119/1 -> Mux26/9
  Data Type Conversion120/1 -> Mux26/8
  Drive 2/2(rotor_tics) -> [lAr]
  Drive 10/2(rotor_tics) -> [rAr]
  [rAState] -> Mux/2
  [rBState] -> Mux/1
  [lBState] -> Mux/3
  [lAState] -> Mux/4
  [rHState] -> Mux/5
  [lHState] -> Mux/6
  Mux/1 -> medulla_states/1
  Box 7/2(ErrorFlags) -> [rAErrorFlags]
  [rBErrorFlags] -> Mux7/1
  [imuErrorFlags] -> Mux7/7
  [lHErrorFlags] -> Mux7/6
  [rHErrorFlags] -> Mux7/5
  [lAErrorFlags] -> Mux7/4
  [lBErrorFlags] -> Mux7/3
  [rAErrorFlags] -> Mux7/2
  Data Type Conversion121/1 -> motor_temperatures/1(u)
  Mux17/1 -> Data Type Conversion121/1
  Mux21/1 -> [rBTherms]
  Mux27/1 -> [rATherms]
  Mux31/1 -> [rHTherms]
  Mux32/1 -> [lBTherms]
  Mux33/1 -> [lATherms]
  Mux34/1 -> [lHTherms]
  [rBTherms] -> Mux17/1
  [rATherms] -> Mux17/2
  [lBTherms] -> Mux17/3
  [lATherms] -> Mux17/4
  [rHTherms] -> Mux17/5
  [lHTherms] -> Mux17/6
  FakeLogicVoltage/1 -> Mux35/7
  Mux35/1 -> logic_voltages/1
  [rBLogicVoltage] -> Mux35/1
  [lHLogicVoltage] -> Mux35/6
  [rHLogicVoltage] -> Mux35/5
  [lALogicVoltage] -> Mux35/4
  [lBLogicVoltage] -> Mux35/3
  [rALogicVoltage] -> Mux35/2
  [rAMotorVoltage] -> Mux36/2
  [rBMotorVoltage] -> Mux36/1
  [lBMotorVoltage] -> Mux36/3
  [lAMotorVoltage] -> Mux36/4
  [rHMotorVoltage] -> Mux36/5
  [lHMotorVoltage] -> Mux36/6
  Mux36/1 -> motor_voltages/1
  Box 4/10(Counter) -> Box 4/2(MedullaCounter), Data Type Conversion119/1
  Box 8/3(LegEncoder) -> [rBLegTicks]
  Box 8/4(MotorEncoder) -> [rBMotorTicks]
  Box 8/5(LegEncoderTimestamp) -> [rBLegTs]
  Box 8/6(MotorEncoderTimestamp) -> [rBMotorTs]
  Box 7/6(MotorEncoderTimestamp) -> [rAMotorTs]
  Box 7/5(LegEncoderTimestamp) -> [rALegTs]
  Box 7/4(MotorEncoder) -> [rAMotorTicks]
  Box 7/3(LegEncoder) -> [rALegTicks]
  Box 5/3(LegEncoder) -> [lBLegTicks]
  Box 5/4(MotorEncoder) -> [lBMotorTicks]
  Box 5/5(LegEncoderTimestamp) -> [lBLegTs]
  Box 5/6(MotorEncoderTimestamp) -> [lBMotorTs]
  Box 6/3(LegEncoder) -> [lALegTicks]
  Box 6/4(MotorEncoder) -> [lAMotorTicks]
  Box 6/5(LegEncoderTimestamp) -> [lALegTs]
  Box 6/6(MotorEncoderTimestamp) -> [lAMotorTs]
  [lBCounter] -> Box 5/2(MedullaCounter)
  [rBCounter] -> Box 8/2(MedullaCounter)
  [rACounter] -> Box 7/2(MedullaCounter)
  [lACounter] -> Box 6/2(MedullaCounter)
  Box 11/12(Counter) -> [rHCounter]
  [rHCounter] -> Box 11/2(MedullaCounter)
  Box 11/3(HipEncoder) -> [rHAbsTicks]
  Box 11/4(IncEncoder) -> [rHIncTicks]
  Box 11/5(HipEncoderTimestamp) -> [rHAbsTs]
  Box 11/6(IncEncoderTimestamp) -> [rHIncTs]
  Box 1/12(Counter) -> [lHCounter]
  [lHCounter] -> Box 1/2(MedullaCounter)
  Box 1/3(HipEncoder) -> [lHAbsTicks]
  Box 1/4(IncEncoder) -> [lHIncTicks]
  Box 1/5(HipEncoderTimestamp) -> [lHAbsTs]
  Box 1/6(IncEncoderTimestamp) -> [lHIncTs]
  RB Leg Encoder/3 -> Terminator4/1
  [rBLegTicks] -> RB Leg Encoder/1
  [rBCounter] -> RB Leg Encoder/2
  [rBLegTs] -> RB Leg Encoder/3
  RB Leg Encoder/1 -> [rBLegQ]
  RB Leg Encoder/2 -> [rBLegDQ]
  FakeBoom/1 -> [BoomEncs]
  raw_encoder_signals/1 -> Terminator5/1
  Mux1/1 -> raw_encoder_signals/1
  qinc_signals/1 -> inc_pos/1
  dqinc_signals/1 -> inc_vel/1
  Mux3/1 -> qinc_signals/1
  Mux4/1 -> dqinc_signals/1
  Mux5/1 -> [LegQ]
  Mux6/1 -> [LegDQ]
  q_signals/1 -> Terminator8/1
  dq_signals/1 -> Terminator10/1
  Mux8/1 -> q_signals/1
  Mux9/1 -> dq_signals/1
  [LegQ] -> Mux8/1
  [LegDQ] -> Mux9/1
  Mux10/1 -> q/1
  Mux15/1 -> dq/1
  [LegQ] -> Mux10/1
  [LegDQ] -> Mux15/1
  [BoomEncs] -> Mux10/3
  Mux16/1 -> [HipIncQ]
  Mux18/1 -> [HipIncDQ]
  [HipIncQ] -> Mux3/5
  [HipIncDQ] -> Mux4/5
  [rBLegQ] -> Mux5/1
  [rBLegDQ] -> Mux6/1
  [rBMotorTicks] -> RB Motor Encoder/1
  [rBCounter] -> RB Motor Encoder/2
  [rBMotorTs] -> RB Motor Encoder/3
  RB Motor Encoder/1 -> [rBMotorQ]
  RB Motor Encoder/2 -> [rBMotorDQ]
  RB Motor Encoder/3 -> RB Rotor Encoder/3
  [rBMotorQ] -> Mux5/2
  [rBMotorDQ] -> Mux6/2
  [rBMotorQ] -> RB Rotor Encoder/2
  [rBr] -> RB Rotor Encoder/1
  RB Rotor Encoder/1 -> [rBRotorQ]
  RB Rotor Encoder/2 -> [rBRotorDQ]
  [rBRotorQ] -> Mux3/1
  [rBRotorDQ] -> Mux4/1
  [HipIncQ] -> Mux10/2
  [HipIncDQ] -> Mux15/2
  [BoomEncs] -> Mux15/3
  [BoomEncs] -> Mux8/4
  [BoomEncs] -> Mux9/4
  RA Leg Encoder/3 -> Terminator11/1
  [rALegTicks] -> RA Leg Encoder/1
  [rACounter] -> RA Leg Encoder/2
  [rALegTs] -> RA Leg Encoder/3
  RA Leg Encoder/1 -> [rALegQ]
  RA Leg Encoder/2 -> [rALegDQ]
  [rAMotorTicks] -> RA Motor Encoder/1
  [rACounter] -> RA Motor Encoder/2
  [rAMotorTs] -> RA Motor Encoder/3
  RA Motor Encoder/1 -> [rAMotorQ]
  RA Motor Encoder/2 -> [rAMotorDQ]
  RA Motor Encoder/3 -> RA Rotor Encoder/3
  [rAMotorQ] -> RA Rotor Encoder/2
  RA Rotor Encoder/1 -> [rARotorQ]
  RA Rotor Encoder/2 -> [rARotorDQ]
  [rAr] -> RA Rotor Encoder/1
  [rAMotorDQ] -> Mux6/4
  [rALegDQ] -> Mux6/3
  [rAMotorQ] -> Mux5/4
  [rALegQ] -> Mux5/3
  [rARotorQ] -> Mux3/2
  [rARotorDQ] -> Mux4/2
  LB Leg Encoder/3 -> Terminator14/1
  [lBLegTicks] -> LB Leg Encoder/1
  [lBCounter] -> LB Leg Encoder/2
  [lBLegTs] -> LB Leg Encoder/3
  LB Leg Encoder/1 -> [lBLegQ]
  LB Leg Encoder/2 -> [lBLegDQ]
  [lBMotorTicks] -> LB Motor Encoder/1
  [lBCounter] -> LB Motor Encoder/2
  [lBMotorTs] -> LB Motor Encoder/3
  LB Motor Encoder/1 -> [lBMotorQ]
  LB Motor Encoder/2 -> [lBMotorDQ]
  LB Motor Encoder/3 -> LB Rotor Encoder/3
  [lBMotorQ] -> LB Rotor Encoder/2
  [lBr] -> LB Rotor Encoder/1
  LB Rotor Encoder/1 -> [lBRotorQ]
  LB Rotor Encoder/2 -> [lBRotorDQ]
  LA Leg Encoder/3 -> Terminator13/1
  [lALegTicks] -> LA Leg Encoder/1
  [lACounter] -> LA Leg Encoder/2
  [lALegTs] -> LA Leg Encoder/3
  LA Leg Encoder/1 -> [lALegQ]
  LA Leg Encoder/2 -> [lALegDQ]
  [lAMotorTicks] -> LA Motor Encoder/1
  [lACounter] -> LA Motor Encoder/2
  [lAMotorTs] -> LA Motor Encoder/3
  LA Motor Encoder/1 -> [lAMotorQ]
  LA Motor Encoder/2 -> [lAMotorDQ]
  [lBLegQ] -> Mux5/5
  [lBMotorQ] -> Mux5/6
  [lALegQ] -> Mux5/7
  [lAMotorQ] -> Mux5/8
  [lBLegDQ] -> Mux6/5
  [lBMotorDQ] -> Mux6/6
  [lALegDQ] -> Mux6/7
  [lAMotorDQ] -> Mux6/8
  [lBRotorQ] -> Mux3/3
  [lARotorQ] -> Mux3/4
  [lBRotorDQ] -> Mux4/3
  [lARotorDQ] -> Mux4/4
  [rHAbsTicks] -> RH Absolute Encoder/1
  [rHCounter] -> RH Absolute Encoder/2
  [rHAbsTs] -> RH Absolute Encoder/3
  RH Absolute Encoder/1 -> [rHAbsQ]
  RH Absolute Encoder/2 -> [rHAbsDQ]
  RH Absolute Encoder/3 -> RH Incremental Encoder/5
  [rHIncTicks] -> RH Incremental Encoder/1
  [rHCounter] -> RH Incremental Encoder/2
  [rHIncTs] -> RH Incremental Encoder/3
  [rHAbsQ] -> RH Incremental Encoder/4
  RH Incremental Encoder/1 -> [rHIncQ]
  RH Incremental Encoder/2 -> [rHIncDQ]
  [rHIncQ] -> Mux16/1
  [rHIncDQ] -> Mux18/1
  [lHIncDQ] -> Mux18/2
  [lHIncQ] -> Mux16/2
  [rHAbsQ] -> Mux8/2
  [lHAbsQ] -> Mux8/3
  [rHAbsDQ] -> Mux9/2
  [lHAbsDQ] -> Mux9/3
  [lHAbsTicks] -> LH Absolute Encoder/1
  [lHCounter] -> LH Absolute Encoder/2
  [lHAbsTs] -> LH Absolute Encoder/3
  LH Absolute Encoder/1 -> [lHAbsQ]
  LH Absolute Encoder/2 -> [lHAbsDQ]
  LH Absolute Encoder/3 -> LH Incremental Encoder/5
  [lHIncTicks] -> LH Incremental Encoder/1
  [lHCounter] -> LH Incremental Encoder/2
  [lHIncTs] -> LH Incremental Encoder/3
  [lHAbsQ] -> LH Incremental Encoder/4
  LH Incremental Encoder/1 -> [lHIncQ]
  LH Incremental Encoder/2 -> [lHIncDQ]
  Data Type Conversion1/1 -> Mux1/1
  [rBLegTicks] -> Data Type Conversion1/1
  [rBMotorTicks] -> Data Type Conversion3/1
  Data Type Conversion5/1 -> Mux1/3
  Data Type Conversion3/1 -> Mux1/2
  Data Type Conversion6/1 -> Mux1/4
  [rALegTicks] -> Data Type Conversion5/1
  [rAMotorTicks] -> Data Type Conversion6/1
  Data Type Conversion8/1 -> Mux1/6
  Data Type Conversion7/1 -> Mux1/5
  Data Type Conversion9/1 -> Mux1/7
  Data Type Conversion10/1 -> Mux1/8
  [lBLegTicks] -> Data Type Conversion7/1
  [lBMotorTicks] -> Data Type Conversion8/1
  [lALegTicks] -> Data Type Conversion9/1
  [lAMotorTicks] -> Data Type Conversion10/1
  Data Type Conversion12/1 -> Mux1/9
  [rHAbsTicks] -> Data Type Conversion12/1
  [rHIncTicks] -> Data Type Conversion13/1
  [lHAbsTicks] -> Data Type Conversion14/1
  [lHIncTicks] -> Data Type Conversion11/1
  Data Type Conversion13/1 -> Mux1/10
  Data Type Conversion14/1 -> Mux1/11
  Data Type Conversion11/1 -> Mux1/12
  [BoomEncs] -> Mux1/13
  LA Motor Encoder/3 -> LA Rotor Encoder/3
  [lAMotorQ] -> LA Rotor Encoder/2
  [lAr] -> LA Rotor Encoder/1
  LA Rotor Encoder/1 -> [lARotorQ]
  LA Rotor Encoder/2 -> [lARotorDQ]
  Hottest Motor/1 -> If Hotter than Maximum/1
  If Hotter than Maximum/1 -> Thermal_Indicator/1
  Thermal_Indicator/1 -> Terminator1/1
  [rAMotorVoltage] -> Data Type Conversion15/1
  Data Type Conversion15/1 -> battery_ADC_to_volts/1(u)
  battery_ADC_to_volts/1(volt) -> battery_voltage/1
  Box 5/18(BatteryCurrent) -> [BatteryCurrent]
  [BatteryCurrent] -> Data Type Conversion16/1
  Data Type Conversion16/1 -> battery_ADC_to_current/1(u)
  battery_ADC_to_current/1(amps) -> battery_current/1
  Demux2/1 -> [RightBackVelocityCmd]
  Demux2/2 -> [RightFrontVelocityCmd]
  Demux2/3 -> [LeftBackVelocityCmd]
  Demux2/4 -> [LeftFrontVelocityCmd]
  Enable Elmo Velocity Mode [true/false] x4/1 -> 1kHz to 2kHz4/1
  Demux3/1 -> [RightBackVelocityMode]
  Demux3/2 -> [RightFrontVelocityMode]
  Demux3/3 -> [LeftBackVelocityMode]
  Demux3/4 -> [LeftFrontVelocityMode]
  [RightFrontVelocityMode] -> Drive 10/3(EnableVelocityMode)
  [RightFrontVelocityCmd] -> Drive 10/2(VelocityCmd)
  [RightBackVelocityCmd] -> Drive 9/2(VelocityCmd)
  [RightBackVelocityMode] -> Drive 9/3(EnableVelocityMode)
  [LeftFrontVelocityMode] -> Drive 2/3(EnableVelocity Mode)
  [LeftFrontVelocityCmd] -> Drive 2/2(VelocityCmd)
  [LeftBackVelocityCmd] -> Drive 3/2(VelocityCmd)
  [LeftBackVelocityMode] -> Drive 3/3(EnableVelocityMode)
  Drive 2/4(Velocity Actual Value) -> [LeftFrontElmoVelocity]
  Drive 3/4(Velocity Actual Value) -> [LeftBackElmoVelocity]
  Drive 10/4(Velocity Actual Value) -> [RightFrontElmoVelocity]
  Drive 9/4(Velocity Actual Value) -> [RightBackElmoVelocity]
  [RightBackElmoVelocity] -> Mux19/1
  [RightFrontElmoVelocity] -> Mux19/2
  [LeftBackElmoVelocity] -> Mux19/3
  [LeftFrontElmoVelocity] -> Mux19/4
  Mux19/1 -> Mux29/1
  Elmo Velocity Commands [rad/s] x4/1 -> Convert geared rad/s to rotor cnts/s/1(in)
  Convert geared rad/s to rotor cnts/s/1(out) -> 1kHz to 2kHz5/1
  Measured/1 -> Elmo Measured Velocity/1
  Mux2/1 -> "Unit Delay "/1
  Drive 2/6(CurrentCmd) -> [LeftFrontElmoCurrentCmd]
  Drive 10/6(CurrentCmd) -> [RightFrontElmoCurrentCmd]
  Drive 9/6(CurrentCmd) -> [RightBackElmoCurrentCmd]
  Drive 3/6(CurrentCmd) -> [LeftBackElmoCurrentCmd]
  Box 1/13(CurrentCmd) -> [LeftLateralCurrentCmd]
  Box 11/13(CurrentCmd) -> [RightLateralCurrentCmd]
  [RightBackElmoCurrentCmd] -> Mux2/1
  [RightFrontElmoCurrentCmd] -> Mux2/2
  [LeftBackElmoCurrentCmd] -> Mux2/3
  [LeftFrontElmoCurrentCmd] -> Mux2/4
  [RightLateralCurrentCmd] -> Mux20/1
  [LeftLateralCurrentCmd] -> Mux20/2
  Mux20/1 -> Unit Delay 1/1
  "Unit Delay "/1 -> Elmo Current Commands/1
  Unit Delay 1/1 -> Lateral Current Commands/1
  [RightBackElmoCurrentDemand] -> Mux22/1
  [RightFrontElmoCurrentDemand] -> Mux22/2
  [LeftBackElmoCurrentDemand] -> Mux22/3
  [LeftFrontElmoCurrentDemand] -> Mux22/4
  Mux22/1 -> Conversion1/1(Elmo Current)
  Conversion1/1(Torque) -> Elmo Demanded Torque/1
  Drive 2/7(Elmo Torque Demand) -> [LeftFrontElmoCurrentDemand]
  Drive 3/7(Elmo Torque Demand) -> [LeftBackElmoCurrentDemand]
  Drive 10/7(Elmo Torque Demand) -> [RightFrontElmoCurrentDemand]
  Drive 9/7(Elmo Torque Demand) -> [RightBackElmoCurrentDemand]
  Drive 2/8(Error Code) -> [LeftFrontElmoErrorCode]
  Drive 3/8(Error Code) -> [LeftBackElmoErrorCode]
  Drive 10/8(Error Code) -> [RightFrontElmoErrorCode]
  Drive 9/8(Error Code) -> [RightBackElmoErrorCode]
  [RightBackElmoErrorCode] -> Mux23/1
  [RightFrontElmoErrorCode] -> Mux23/2
  [LeftBackElmoErrorCode] -> Mux23/3
  [LeftFrontElmoErrorCode] -> Mux23/4
  Mux23/1 -> Elmo Error Codes/1
  Drive 2/5(Velocity Demand Value) -> [LeftFrontElmoVelocityDemand]
  Drive 10/5(Velocity Demand Value) -> [RightFrontElmoVelocityDemand]
  Drive 3/5(Velocity Demand Value) -> [LeftBackElmoVelocityDemand]
  Drive 9/5(Velocity Demand Value) -> [RightBackElmoVelocityDemand]
  [RightBackElmoVelocityDemand] -> Mux24/1
  [RightFrontElmoVelocityDemand] -> Mux24/2
  [LeftBackElmoVelocityDemand] -> Mux24/3
  [LeftFrontElmoVelocityDemand] -> Mux24/4
  Mux24/1 -> Mux29/2
  Convert rotor cnt/s to geared rad/s/1(out) -> Demanded/1, Measured/1
  Mux29/1 -> Convert rotor cnt/s to geared rad/s/1(in)
  Demanded/1 -> Elmo Demanded Velocity/1
  1kHz to 2kHz5/1 -> Demux2/1
  1kHz to 2kHz4/1 -> Demux3/1
  1kHz to 2kHz/1 -> Drive 2/1(MotorCmd)
  1kHz to 2kHz3/1 -> Drive 3/1(MotorCmd)
  1kHz to 2kHz2/1 -> Drive 9/1(MotorCmd)
  1kHz to 2kHz1/1 -> Drive 10/1(MotorCmd)

== system atrias_system_4khz/Ramp Velocity Commands ==
  note: For GUI
  is_run_cmd : Inport  OutDataTypeStr=boolean  PortDimensions=1
  velocity_cmd [rad/s] x4 : Inport  Port=2
  Constant : Constant  Value=0.1
  Current Time : Clock
  Enabled time : Sum  Inputs=-+
  Hold Start Time : Subsystem  TreatAsAtomicUnit=on
  NOT : Logic  Operator=NOT  IconShape=distinctive  AllPortsSameDT=off  OutDataTypeStr=boolean
  Ramp Rate (Units/sec) : Gain  Gain=1/4
  Scaling Factor : Saturate  UpperLimit=1  LowerLimit=0
  Startup Ramp : Product
  Sum : Sum  Inputs=|-+
  Terminator : Terminator
  is_start_done_cmp : RelationalOperator  Operator=>  OutDataTypeStr=boolean  RndMeth=Nearest
  velocity_cmd_scaled [rad/s] x4 : Outport  OutDataTypeStr=double  PortDimensions=4
  wires:
  is_start_done_cmp/1 -> Terminator/1
  Sum/1 -> is_start_done_cmp/1
  velocity_cmd [rad/s] x4/1 -> Startup Ramp/2
  Startup Ramp/1 -> velocity_cmd_scaled [rad/s] x4/1
  Scaling Factor/1 -> Startup Ramp/1, is_start_done_cmp/2
  Ramp Rate (Units/sec)/1 -> Sum/2, Scaling Factor/1
  Enabled time/1 -> Ramp Rate (Units/sec)/1
  Hold Start Time/1(Time Out) -> Enabled time/1
  Current Time/1 -> Hold Start Time/1(Time In), Enabled time/2
  is_run_cmd/1 -> NOT/1
  NOT/1 -> Hold Start Time/Enable
  Constant/1 -> Sum/1

== system atrias_system_4khz/Start Controller ==
  note: For GUI
  note: Input Order:
      |
      | backR
      | frontR
      | latR
      | backL
      | frontL
      | latL
  is_run_cmd : Inport  OutDataTypeStr=boolean  PortDimensions=1
  tau_cmd_in [Nm] x6 : Inport  Port=2
  Current Time : Clock
  Enabled time : Sum  Inputs=-+
  Hold Start Time : Subsystem  TreatAsAtomicUnit=on
  Lateral Motor Saturation : Saturate  UpperLimit=HIP_MTR_MAX_TORQUE  LowerLimit=-HIP_MTR_MAX_TORQUE
      settings: AttributesFormatString=Top: %<UpperLimit>\nBottom: %<LowerLimit>
  NOT : Logic  Operator=NOT  IconShape=distinctive  AllPortsSameDT=off  OutDataTypeStr=boolean
  Ramp Rate (Units/sec) : Gain  Gain=.25
  Sagittal Motor Saturation : Saturate  UpperLimit=LEG_MTR_MAX_TORQUE  LowerLimit=-LEG_MTR_MAX_TORQUE
      settings: AttributesFormatString=Top: %<UpperLimit>\nBottom: %<LowerLimit>
  Scaling Factor : Saturate  UpperLimit=1  LowerLimit=0
  Selector : Selector  InputPortWidth=6  IndexOptions=Index vector (dialog)  Indices=[1 2 4 5 6 3]  OutputSizes=1
  Selector1 : Selector  InputPortWidth=6  IndexOptions=Index vector (dialog)  Indices=[1 2 3 4]  OutputSizes=1
  Selector2 : Selector  InputPortWidth=6  IndexOptions=Index vector (dialog)  Indices=[5 6]  OutputSizes=1
  Separated to Tau : Selector  InputPortWidth=6  IndexOptions=Index vector (dialog)  Indices=[1 2 6 3 4 5]  OutputSizes=1
  Startup Tau Ramp : Product
  Sum : Sum  Inputs=|-+
  Terminator : Terminator
  Vector Concatenate : Concatenate
  is_start_done_cmp : RelationalOperator  Operator=>  OutDataTypeStr=boolean  RndMeth=Nearest
  tau_cmd_out [Nm] x6 : Outport  OutDataTypeStr=double  PortDimensions=6
  wires:
  NOT/1 -> Hold Start Time/Enable
  is_run_cmd/1 -> NOT/1
  Current Time/1 -> Enabled time/2, Hold Start Time/1(Time In)
  Hold Start Time/1(Time Out) -> Enabled time/1
  Enabled time/1 -> Ramp Rate (Units/sec)/1
  Ramp Rate (Units/sec)/1 -> Scaling Factor/1, Sum/2
  Scaling Factor/1 -> is_start_done_cmp/2, Startup Tau Ramp/1
  Startup Tau Ramp/1 -> tau_cmd_out [Nm] x6/1
  Selector2/1 -> Lateral Motor Saturation/1  "lateral"
  Selector1/1 -> Sagittal Motor Saturation/1  "sagittal"
  tau_cmd_in [Nm] x6/1 -> Selector/1
  Selector/1 -> Selector1/1, Selector2/1
  Sagittal Motor Saturation/1 -> Vector Concatenate/1
  Lateral Motor Saturation/1 -> Vector Concatenate/2
  Vector Concatenate/1 -> Separated to Tau/1
  Separated to Tau/1 -> Startup Tau Ramp/2
  Sum/1 -> is_start_done_cmp/1
  is_start_done_cmp/1 -> Terminator/1
